simulink model "demoUSBserialFrame"  (R2016a)
settings: Solver=FixedStepAuto  StartTime=0.0  StopTime=inf  FixedStep=0.1  RelTol=1e-3
libraries: frdmKL25Z x2, frdmkl25zlib x1
settings Model: SimulationMode=external  ExtModeTrigDuration=5  Creator=user  LastModifiedBy=user
settings OptimizationCC: OptimizeModelRefInitCode=on  LifeSpan=1  MaxStackSize=64
settings HardwareCC: ProdBitPerPointer=32  ProdLargestAtomicInteger=Long  ProdLargestAtomicFloat=Double  ProdWordSize=32  ProdHWDeviceType=ARM Compatible->ARM Cortex
settings RTWCC: SystemTargetFile=ert.tlc  HardwareBoard=Freescale FRDM-KL25Z  TemplateMakefile=ert_default_tmf  GenerateReport=on  Toolchain=GNU Tools for ARM Embedded Processors  IncludeHyperlinkInReport=on  LaunchReport=on  GenerateTraceInfo=on  GenerateTraceReport=on  GenerateTraceReportSl=on  GenerateTraceReportSf=on  GenerateTraceReportEml=on
settings CodeAppCC: ForceParamTrailComments=on  IgnoreCustomStorageClasses=off  OperatorAnnotations=on  SimulinkDataObjDesc=on  SFDataObjDesc=on  MATLABFcnDesc=on  InsertBlockDesc=on  MATLABSourceComments=on

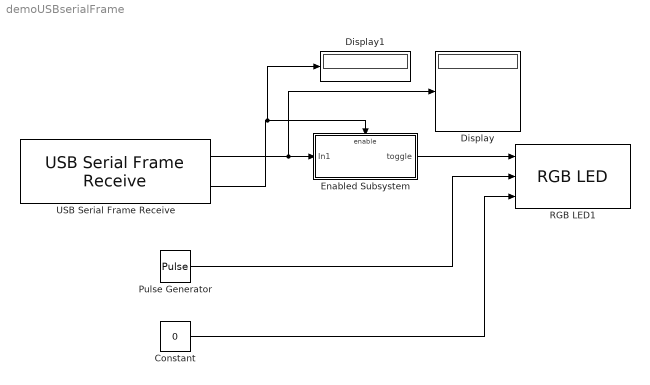
== system demoUSBserialFrame ==
  Constant : Constant  Value=0
  Display : Display
  Display1 : Display
  Enabled Subsystem : Subsystem  TreatAsAtomicUnit=on
  Pulse Generator : DiscretePulseGenerator  Amplitude=100
  RGB LED1 : frdmkl25zlib/RGB LED
  USB Serial Frame Receive : frdmKL25Z/USB Serial Frame Receive  SOFbyte=254  EOFbyte=255  msgLen=10  SimulateUsing=Code generation
  wires:
  USB Serial Frame Receive/1 -> Display/1, Enabled Subsystem/1(In1)
  USB Serial Frame Receive/2 -> Display1/1, Enabled Subsystem/Enable
  Enabled Subsystem/1(toggle) -> RGB LED1/1
  Pulse Generator/1 -> RGB LED1/2
  Constant/1 -> RGB LED1/3

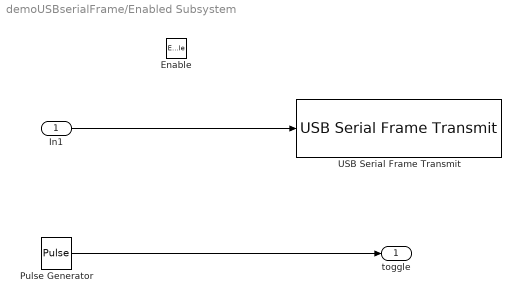
== system demoUSBserialFrame/Enabled Subsystem ==
  In1 : Inport
  Enable : EnablePort
  Pulse Generator : DiscretePulseGenerator  Amplitude=100  SampleTime=-1
  USB Serial Frame Transmit : frdmKL25Z/USB Serial Frame Transmit  SOFbyte=254  EOFbyte=255  SimulateUsing=Code generation
  toggle : Outport
  wires:
  In1/1 -> USB Serial Frame Transmit/1
  Pulse Generator/1 -> toggle/1
